simulink model "GNC_system"  (R2020b)
settings: Solver=VariableStepAuto  StartTime=0.0  StopTime=100  RelTol=1e-3
values from neighbouring files (symbols this model uses):
  A = [-1.064 1.000; 290.26 0.00]    [GNC.m]
  azimuth_ang = azimuth(lat_init,long_init,lat_target*180/pi,long_target*180/pi)    [GNC.m]
  B = [-0.25; -331.40]    [GNC.m]
  C = [-123.34 0; 0 1]    [GNC.m]
  D = [-13.51; 0]    [GNC.m]
  dT1 = 0.75    [GNC.m]
  dT2 = 0.25    [GNC.m]
  elev_init = 10000    [GNC.m]
  elev_target = 0    [GNC.m]
  G = eye(length(A(1,:)))    [GNC.m]
  lat_init = 34.2329    [GNC.m]
  lat_obs = 34.61916*pi/180    (= 0.604218326275)    [GNC.m]
  lat_target = 34.6588*pi/180    (= 0.60491017479)    [GNC.m]
  long_init = -119.4573    [GNC.m]
  long_obs = -118.8429*pi/180    (= -2.07419989762)    [GNC.m]
  long_target = -118.769745*pi/180    (= -2.072923102)    [GNC.m]
  q_bar = diag(0.000015*ones(1,length(G(1,:))))    [GNC.m]
  r_bar = diag(0.001*ones(1,length(G(1,:))))    [GNC.m]
  V = 1021.08    [GNC.m]
undefined symbols (not defined in the file or in its folder): Earth, K, L, WGS84
libraries: simulink x3, aerolibtransform2 x1, aerolibfltsims x1, pid_lib x1
settings Model: PacingRate=5  Creator=surya  LastModifiedBy=surya

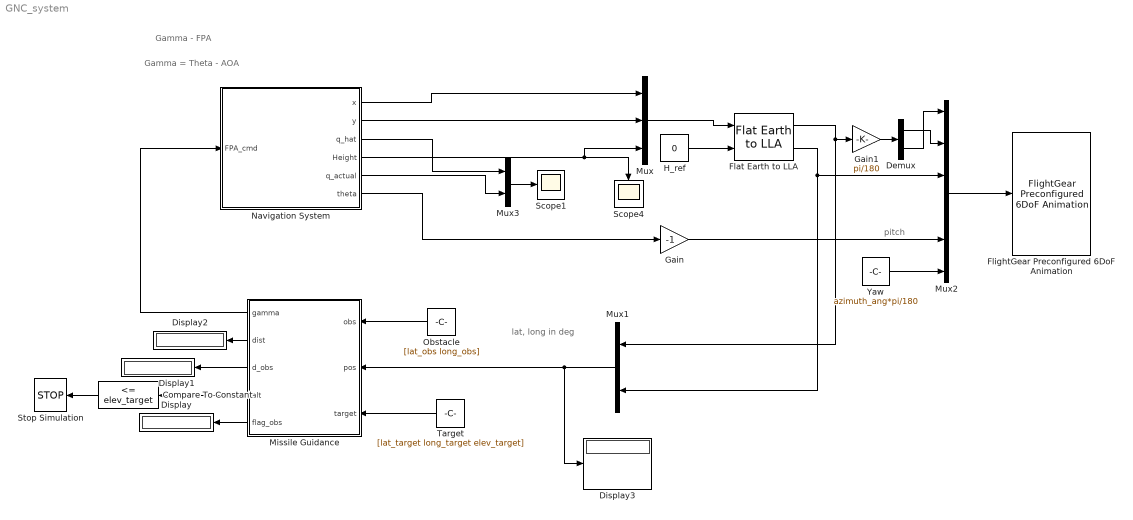
== system GNC_system ==
  note: pitch
  note: lat, long in deg
  note: Gamma - FPA
  note: Gamma = Theta - AOA
  Compare To Constant : simulink/Logic and Bit Operations/Compare To Constant  relop=<=  const=elev_target  OutDataTypeStr=boolean
  Demux : Demux  Outputs=2
  Display{,1..3} (4 alike) : Display
  Flat Earth to LLA : aerolibtransform2/Flat Earth to LLA  units=Metric (MKS)  ptype=Earth (WGS84)  F=1/298.257223563  R=6378137  refPosPort=off  LL0=[lat_init long_init]  psi=azimuth_ang
  FlightGear Preconfigured 6DoF Animation : aerolibfltsims/FlightGear Preconfigured 6DoF Animation  xFlightGearVersion=v2019.1  DestinationIpAddress=127.0.0.1  DestinationPort=5502  SampleTime=1/30  packetVersion=24
  Gain : Gain  Gain=-1
  Gain1 : Gain  Gain=pi/180
  H_ref : Constant  Value=0
  Missile Guidance : MATLAB Function  TreatAsAtomicUnit=on
  Mux : Mux  Inputs=3
  Mux1 : Mux  Inputs=2
  Mux2 : Mux  Inputs=6
  Mux3 : Mux  Inputs=2
  Navigation System : Subsystem
  Obstacle : Constant  Value=[lat_obs long_obs]
  Scope1 : Scope
  Scope4 : Scope
  Stop Simulation : Stop
  Target : Constant  Value=[lat_target long_target elev_target]
  Yaw : Constant  Value=azimuth_ang*pi/180
  wires:
  Mux/1 -> Flat Earth to LLA/1
  H_ref/1 -> Flat Earth to LLA/2
  Obstacle/1 -> Missile Guidance/1(obs)
  Target/1 -> Missile Guidance/3(target)
  Flat Earth to LLA/1 -> Gain1/1, Mux1/1
  Flat Earth to LLA/2 -> Mux1/2, Mux2/3
  Compare To Constant/1 -> Stop Simulation/1
  Missile Guidance/5(flag_obs) -> Display/1
  Missile Guidance/3(d_obs) -> Display1/1
  Missile Guidance/2(dist) -> Display2/1
  Missile Guidance/4(alt) -> Compare To Constant/1
  Mux1/1 -> Display3/1, Missile Guidance/2(pos)
  Navigation System/4(Height) -> Scope4/1, Mux/3
  Missile Guidance/1(gamma) -> Navigation System/1(FPA_cmd)
  Navigation System/1(x) -> Mux/1
  Navigation System/2(y) -> Mux/2
  Mux2/1 -> FlightGear Preconfigured 6DoF Animation/1
  Demux/2 -> Mux2/1
  Demux/1 -> Mux2/2
  Mux3/1 -> Scope1/1
  Navigation System/3(q_hat) -> Mux3/1
  Navigation System/5(q_actual) -> Mux3/2
  Navigation System/6(theta) -> Gain/1
  Gain/1 -> Mux2/5
  Gain1/1 -> Demux/1
  Yaw/1 -> Mux2/6

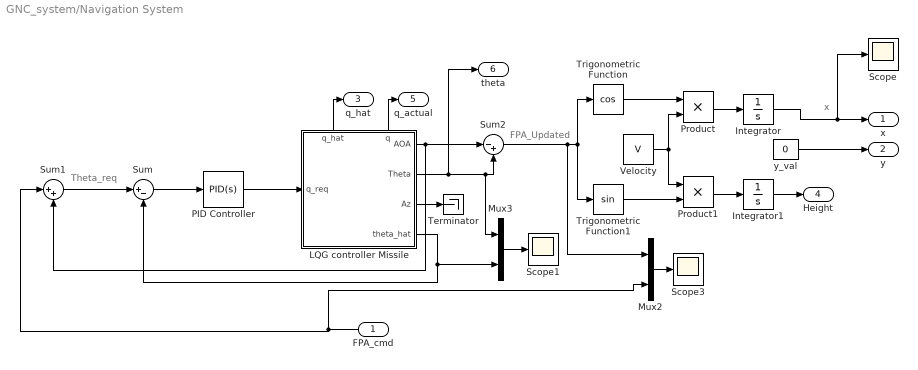
== system GNC_system/Navigation System ==
  note: x
  note: FPA_Updated
  note: Theta_req
  FPA_cmd : Inport
  Integrator : Integrator
  Integrator1 : Integrator  InitialCondition=-elev_init
  LQG controller Missile : Subsystem
      settings: PortSchema="{\"entries\":[{\"content\":{\"sides\":[{\"content\":{\"connectorIds\":[\"In1\"]},\"type\":\"ConnectorPlacement.EquallySpacedRectSide\",\"uuid\":\"9b3f02f4-0603-4cb6-b2b8-26cc0ebf33cc\"},{\"content\":{\"connectorIds\":[\"Out1\",\"Out2\",\"Out3\",\"Out4\"],\"side\":\"RIGHT\"},\"type\":\"ConnectorPlacement.EquallySpacedRectSide\",\"uuid\":\"37295306-7835-4e5a-ae3e-021ba3432403\"},{\"content\":{\"connectorIds\":[\"Out5\",\"Out6\"],\"side\":\"TOP\"},\"type\":\"ConnectorPlacement.EquallySpacedRectSide\",\"uuid\":\"95de3cb4-1f88-4452-9624-98a7345c28e5\"},{\"content\":{\"connectorIds\":[],\"side\":\"HIDDEN\"},\"type\":\"ConnectorPlacement.EquallySpacedRectSide\",\"uuid\":\"00813b65-0a12-4d5b-8b8c-ff569b114e96\"}]},\"type\":\"ConnectorPlacement.EquallySpacedConnector\",\"uuid\":\"5aa4f7f9-c12d-4048-bbb1-e5fab7cad66b\"}],\"packageUris\":[\"http://schema.mathworks.com/mf0/Connector/R2020b\"],\"version\":\"1.0\"}"
  Mux2 : Mux  Inputs=2
  Mux3 : Mux  Inputs=2
  PID Controller : pid_lib/PID Controller  Controller=PID  Form=Parallel  TimeDomain=Continuous-time  UseExternalTs=off  SampleTime=-1  IntegratorMethod=Forward Euler  FilterMethod=Forward Euler  ControllerParametersSource=internal  P=-0.5570607772887  I=-0.059477930454573  D=-0.393140329548918  UseFilter=on  N=72.5130438761651  TunerSelectOption=Transfer Function Based (PID Tuner App)  InitialConditionSource=internal  InitialConditionForIntegrator=0  InitialConditionForFilter=0  DifferentiatorICPrevScaledInput=0  ExternalReset=none  TrackingMode=off  Kt=1  LimitOutput=on  SatLimitsSource=internal  UpperSaturationLimit=0.39  LowerSaturationLimit=-0.39  LinearizeAsGain=on  AntiWindupMode=none  Kb=1  POutMin=[]  POutMax=[]  IOutMin=[]  IOutMax=[]  DOutMin=[]  DOutMax=[]  NOutMin=[]  NOutMax=[]  SumOutMin=[]  SumOutMax=[]  SaturationOutMin=[]  SaturationOutMax=[]  PParamMin=[]  PParamMax=[]  IParamMin=[]  IParamMax=[]  DParamMin=[]  DParamMax=[]  NParamMin=[]  NParamMax=[]  KbParamMin=[]  KbParamMax=[]  KtParamMin=[]  KtParamMax=[]  KbOutMin=[]  KbOutMax=[]  KtOutMin=[]  KtOutMax=[]  IntegratorOutMin=[]  IntegratorOutMax=[]  FilterOutMin=[]  FilterOutMax=[]  SumI1OutMin=[]  SumI1OutMax=[]  SumI2OutMin=[]  SumI2OutMax=[]  SumI3OutMin=[]  SumI3OutMax=[]  SumI4OutMin=[]  SumI4OutMax=[]  SumDOutMin=[]  SumDOutMax=[]  DifferentiatorOutMin=[]  DifferentiatorOutMax=[]  FilterDiffOutCoefMin=[]  FilterDiffOutCoefMax=[]  ReciprocalOutMin=[]  ReciprocalOutMax=[]  SumDenOutMin=[]  SumDenOutMax=[]  SumNumOutMin=[]  SumNumOutMax=[]  DivideOutMin=[]  DivideOutMax=[]  UdiffTsProdOutMin=[]  UdiffTsProdOutMax=[]  NTsProdOutMin=[]  NTsProdOutMax=[]  UintegralTsProdOutMin=[]  UintegralTsProdOutMax=[]  UngainTsProdOutMin=[]  UngainTsProdOutMax=[]  IntegratorContinuousStateAttributes=''  IntegratorStateMustResolveToSignalObject=off  IntegratorRTWStateStorageClass=Auto  FilterContinuousStateAttributes=''  FilterStateMustResolveToSignalObject=off  FilterRTWStateStorageClass=Auto  ParallelPVariant=InternalParameters  IdealPVariant=Disabled  IVariant=InternalParameters  DVariant=InternalParameters  IntegratorVariant=Continuous  SatVariant=Enabled  AWVariant=Passthrough  PCopyVariant=Disabled  TRVariant=Disabled  FdbkBlocksVariant=Forward  IdealPFdbkVariant=Disabled  SatFdbkVariant=Disabled  DerivativeFilterVariant=ContFilter  NVariant=InternalParameters  NCopyVariant=Disabled  FilterICVariant=InternalICsFilter  IntegratorICVariant=InternalICs  ExternalResetVariant=Disabled  TRSumVariant=Passthrough  SumFdbkVariant=Disabled  SumVariant=Sum_PID  TsampFilterVariant=InternalTs  TsampNgainVariant=Passthrough  TsampIntegralVariant=Passthrough  ExternalSaturationOutDataTypeStr=Inherit: Same as second input
  Product : Product
  Product1 : Product
  Scope : Scope
  Scope1 : Scope
  Scope3 : Scope
  Sum : Sum  Inputs=|+-
  Sum1 : Sum  Inputs=|++
  Sum2 : Sum  Inputs=|-+
  Terminator : Terminator
  Trigonometric Function : Trigonometry  Operator=cos
  Trigonometric Function1 : Trigonometry
  Velocity : Constant  Value=V
  y_val : Constant  Value=0
  x : Outport
  y : Outport  Port=2
  q_hat : Outport  Port=3
  Height : Outport  Port=4
  q_actual : Outport  Port=5
  theta : Outport  Port=6
  wires:
  Product1/1 -> Integrator1/1
  Velocity/1 -> Product1/1, Product/2
  PID Controller/1 -> LQG controller Missile/1(q_req)
  LQG controller Missile/6(q) -> q_actual/1
  LQG controller Missile/1(AOA) -> Sum1/2, Sum2/1
  LQG controller Missile/4(theta_hat) -> Mux3/2, Sum/2
  FPA_cmd/1 -> Sum1/1, Mux2/2
  LQG controller Missile/2(Theta) -> theta/1, Mux3/1, Sum2/2
  Product/1 -> Integrator/1
  Sum/1 -> PID Controller/1
  LQG controller Missile/3(Az) -> Terminator/1
  Integrator/1 -> Scope/1, x/1
  Trigonometric Function/1 -> Product/1
  LQG controller Missile/5(q_hat) -> q_hat/1
  Sum1/1 -> Sum/1
  Sum2/1 -> Trigonometric Function1/1, Trigonometric Function/1, Mux2/1
  Trigonometric Function1/1 -> Product1/2
  Mux2/1 -> Scope3/1
  Mux3/1 -> Scope1/1
  Integrator1/1 -> Height/1
  y_val/1 -> y/1

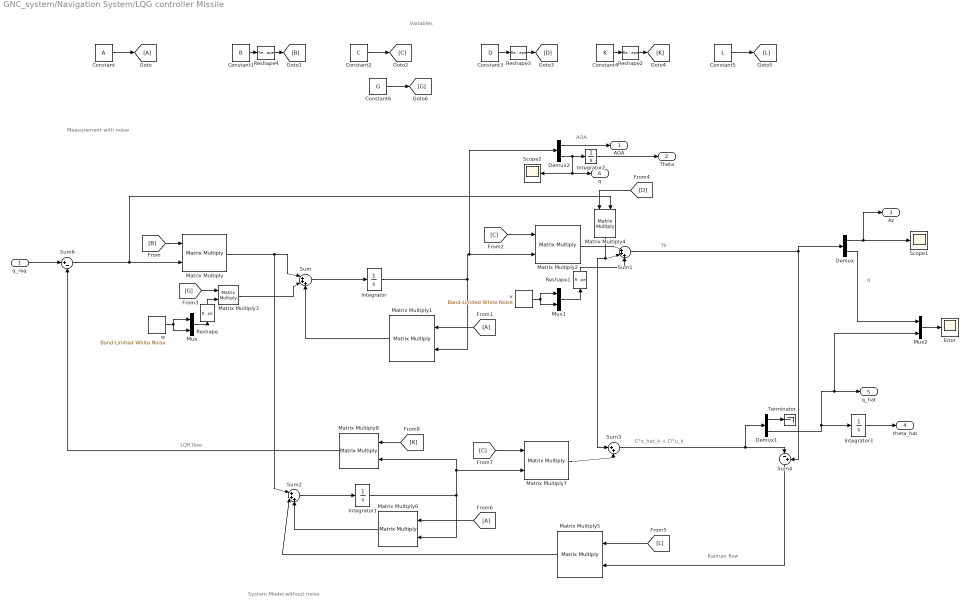
== system GNC_system/Navigation System/LQG controller Missile ==
  note: System Model without noise
  note: Measurement with noise
  note: Kalman flow
  note: LQR flow
  note: AOA
  note: q
  note: Variables
  note: C*x_hat_k + D*u_k
  note: Yk
  q_req : Inport
  Constant : Constant  Value=A
  Constant1 : Constant  Value=B
  Constant2 : Constant  Value=C
  Constant3 : Constant  Value=D
  Constant4 : Constant  Value=K
  Constant5 : Constant  Value=L
  Constant6 : Constant  Value=G
  Demux : Demux  Outputs=2
  Demux1 : Demux  Outputs=2
  Demux2 : Demux  Outputs=2
  Error : Scope
  Integrator{,1..3} (4 alike) : Integrator
  Matrix Multiply{,1..8} (9 alike) : Product  Multiplication=Matrix(*)
  Mux : Mux  Inputs=length(G(1,:))
  Mux1 : Mux  Inputs=length(G(1,:))
  Mux2 : Mux  Inputs=length(G(1,:))
  Reshape : Reshape
  Reshape1 : Reshape  OutputDimensionality=Column vector (2-D)
  Reshape2 : Reshape  OutputDimensionality=Customize  OutputDimensions=[1,2]
  Reshape3 : Reshape  OutputDimensionality=Customize  OutputDimensions=[2,1]
  Reshape4 : Reshape  OutputDimensionality=Customize  OutputDimensions=[2,1]
  Scope1 : Scope
  Scope2 : Scope
  Sum : Sum  Inputs=|+++
  Sum1 : Sum  Inputs=|+++
  Sum2 : Sum  Inputs=|+++
  Sum3 : Sum  Inputs=|++
  Sum4 : Sum  Inputs=|-+
  Sum6 : Sum  Inputs=|+-
  Terminator : Terminator
  v : simulink/Sources/Band-Limited White Noise  Cov=[r_bar(1)*dT2]  Ts=dT2  seed=[23341]
  w : simulink/Sources/Band-Limited White Noise  Cov=[q_bar(1)*dT1]  Ts=dT1  seed=[23341]
  AOA : Outport
  Theta : Outport  Port=2
  Az : Outport  Port=3
  theta_hat : Outport  Port=4
  q_hat : Outport  Port=5
  q : Outport  Port=6
  wires:
  Sum6/1 -> Matrix Multiply4/2, Matrix Multiply/2
  [C] -> Matrix Multiply7/1
  [A] -> Matrix Multiply6/1
  Matrix Multiply4/1 -> Sum3/1, Sum1/2
  [D] -> Matrix Multiply4/1
  Sum/1 -> Integrator/1
  Integrator3/1 -> theta_hat/1
  [B] -> Matrix Multiply/1
  [A] -> Matrix Multiply1/1
  Constant/1 -> [A]
  Matrix Multiply/1 -> Sum2/1, Sum/1
  Reshape2/1 -> [K]
  w/1 -> Mux/2, Mux/1
  Matrix Multiply6/1 -> Sum2/3
  Sum4/1 -> Matrix Multiply5/2
  Sum1/1 -> Sum4/2, Demux/1
  v/1 -> Mux1/2, Mux1/1
  Sum2/1 -> Integrator1/1
  Matrix Multiply7/1 -> Sum3/2
  Integrator1/1 -> Matrix Multiply6/2, Matrix Multiply8/2, Matrix Multiply7/2
  Integrator/1 -> Matrix Multiply1/2, Demux2/1, Matrix Multiply2/2
  Reshape1/1 -> Sum1/3
  Matrix Multiply5/1 -> Sum2/2
  Demux/2 -> Mux2/1
  Demux1/2 -> Mux2/2, q_hat/1, Integrator3/1
  Sum3/1 -> Demux1/1, Sum4/1
  Mux/1 -> Reshape/1
  Demux1/1 -> Terminator/1
  Matrix Multiply2/1 -> Sum1/1
  [G] -> Matrix Multiply3/1
  [C] -> Matrix Multiply2/1
  [K] -> Matrix Multiply8/1
  q_req/1 -> Sum6/1
  Reshape3/1 -> [D]
  Integrator2/1 -> Theta/1
  Constant2/1 -> [C]
  Reshape/1 -> Matrix Multiply3/2
  Matrix Multiply3/1 -> Sum/2
  Demux/1 -> Az/1, Scope1/1
  Mux1/1 -> Reshape1/1
  Reshape4/1 -> [B]
  Matrix Multiply1/1 -> Sum/3
  Matrix Multiply8/1 -> Sum6/2
  Demux2/2 -> Scope2/1, q/1, Integrator2/1
  [L] -> Matrix Multiply5/1
  Demux2/1 -> AOA/1
  Constant5/1 -> [L]
  Constant6/1 -> [G]
  Constant4/1 -> Reshape2/1
  Constant1/1 -> Reshape4/1
  Constant3/1 -> Reshape3/1
  Mux2/1 -> Error/1

== matlab function GNC_system/Missile Guidance ==
  data: obs input; gamma output; pos input; target input; dist output; d_obs output; alt output; flag_obs output
function [gamma, dist, d_obs, alt, flag_obs] = fcn(obs, pos, target)

R = 6400e3;
obs_thres = 3500;  % 3.5km obstacle length threshold
deg_rad = pi/180;

d_lat = target(1) - pos(1)*deg_rad;
d_long = target(2) - pos(2)*deg_rad;
dh = abs(pos(3)-target(3));

haversine = sin(d_lat/2)^2 + cos(target(1))*cos(pos(1)*deg_rad)*sin(d_long/2)^2;
d = 2*R*atan2(sqrt(haversine), sqrt(1-haversine));
dist = sqrt(d^2 + dh^2);

d_lat_obs = obs(1) - pos(1)*deg_rad;
d_long_obs = obs(2) - pos(2)*deg_rad;

haversine_obs = sin(d_lat_obs/2)^2 + cos(obs(1))*cos(pos(1)*deg_rad)*sin(d_long_obs/2)^2;
d_obs = 2*R*atan2(sqrt(haversine_obs), sqrt(1-haversine_obs));

if d_obs <= obs_thres
    flag_obs = 1;
    gamma = 0;
else
    flag_obs = 0;
    gamma = atan(dh/d);
end

alt = pos(3);

end
